simulink model "xpcrs232bindemo"  (Simulink 4.00)
settings: Solver=ode5  StartTime=0.0  StopTime=inf  FixedStep=0.01  RelTol=1e-3
undefined symbols (not defined in the file or in its folder): mrs232
libraries: xpclib x5, simulink3 x1
settings Model: Creator=rroy  LastModifiedBy=rroy  RTWSystemTargetFile=xpctarget.tlc  RTWOptions="-aEnforceIntegerDowncast=0 -aExtMode=1 -aFoldNonRolledExpr=0 -aForceParamTrailComments=0 -aGenerateComments=1 -aIncHierarchyInIds=0 -aInlineInvariantSignals=0 -aInlineParameters=0 -aLocalBlockOutputs=0 -aRL32IRQSourceModifier=\"Timer\" -aRL32LogBufSizeModifier=100000 -aRL32LogTETModifier=1 -aRL32ModeModifier=\"Real-Time\" -aRL32ObjectName=\"tg\" -aRL32ScopeModifier=1 -aRTWVerbose=1 -aRollThreshold=5 -aShowEliminatedStatements=1"  RTWTemplateMakefile=xpc_default_tmf  ExtModeMexFile=ext_xpc  ExtModeArmWhenConnect=off  OptimizeBlockIOStorage=off

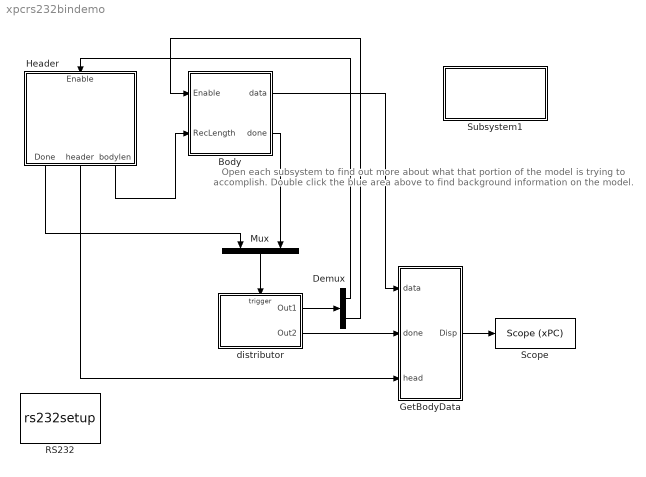
== system xpcrs232bindemo ==
  note: Open each subsystem to find out more
      | about what that portion of the model
      | is trying to accomplish.
      | Double click the blue area above to find
      | background information on the model.
  Body : Subsystem  TreatAsAtomicUnit=on
      settings: RTWFcnNameOpts=Auto  RTWFileNameOpts=Auto
  Demux : Demux  Outputs=2  BusSelectionMode=off
  GetBodyData : Subsystem
      settings: RTWFcnNameOpts=Auto  RTWFileNameOpts=Auto
  Header : Subsystem  Orientation=down  TreatAsAtomicUnit=on
      settings: RTWFcnNameOpts=Auto  RTWFileNameOpts=Auto
  Mux : Mux  Orientation=down  Inputs=2
  "RS232 " : S-Function  AncestorBlock=xpclib/RS232/RS232  InitFcn=mrs232(0);  FunctionName=rs232setup  Parameters=port, baud, dbits, sbits, parity, prot, sbuf, rbuf, 0, istr, iack, iackto, tstr, tack, tackto, initinfo, initackinfo, terminfo, termackinfo  PortCounts=[]  SFunctionModules=''  mask(rs232setup){port=COM1, baud=115200, dbits=8, sbits=1, parity=None, prot=None, sbuf=1024, rbuf=1024, initstruct=[], termstruct=[]}
      mask prompts: baud "Baudrate:"; dbits "Number of Databits:"; sbits "Number of Stopbits:"; prot "Protocol:"; sbuf "Send Buffer Size:"; rbuf "Receive Buffer Size:"; initstruct "Initialization Struct:"; termstruct "Termination Struct:"
      mask help:
      | RS-232
      | Mainboard
      | Setup
      mask init:
      | dmy = '';
      | [istr,iack,dmy,maskdisplay,maskdescription,dmy,dmy,dmy,dmy,initinfo,initackinfo,iackto]=mrs232(2,initstruct,4);
      | [tstr,tack,dmy,maskdisplay,maskdescription,dmy,dmy,dmy,dmy,terminfo,termackinfo,tackto]=mrs232(1,termstruct,4);
      | set_param(gcb,'MaskDisplay',maskdisplay);
      | set_param(gcb,'MaskDescription',maskdescription);
      mask Help: helpview([docroot '/toolbox/xpc/pt_io_block_reference.html#xpcioref'])
      mask StyleString: popup(COM1|COM2|COM3|COM4),popup(115200|57600|38400|19200|9600|4800|2400|1200|600|300|110),popup(8|7),popup(1|2),popup(None|Odd|Even),popup(None|XOn XOff),edit,edit,edit,edit
      mask Display: disp('RS-232\nMainboard\nSetup');
  Scope : xpclib/Misc./Scope (xPC)   scopeno=1  scopetype=Target  viewmode=Numerical  grid=on  ylimits=[0,0]  autostart=on  nosamples=3  noprepostsamples=0  interleave=1  triggermode=FreeRun  triggersignal=1  triggerlevel=0.0  triggerslope=either  triggerscope=1
  Subsystem1 : Subsystem
      settings: OpenFcn=helpview([docroot '\mapfiles\xpc.map'], 'RS232_Binary_Example');  RTWFcnNameOpts=Auto  RTWFileNameOpts=Auto
      mask Display: disp('Double Click\nfor help')
  distributor : Subsystem  TreatAsAtomicUnit=on
      settings: RTWFcnNameOpts=Auto  RTWFileNameOpts=Auto
  wires:
  Body/2(done) -> Mux/2
  Header/3(bodylen) -> Body/2(RecLength)
  distributor/1(Out1) -> Demux/1
  Header/2(header) -> GetBodyData/3(head)
  GetBodyData/1(Disp) -> Scope/1
  Mux/1 -> distributor/Trigger
  Demux/1 -> Header/1(Enable)
  Demux/2 -> Body/1(Enable)
  Body/1(data) -> GetBodyData/1(data)
  distributor/2(Out2) -> GetBodyData/2(done)
  Header/1(Done) -> Mux/1

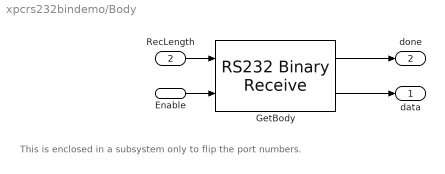
== system xpcrs232bindemo/Body ==
  note: This is enclosed in a subsystem
      | only to flip the port numbers.
  Enable : Inport  Port=1  LatchInput=off
  RecLength : Inport  Port=2  LatchInput=off
  GetBody : xpclib/RS232/Binary Mode/RS232 Binary Receive  port=COM1  width=6  samptime=-1
  data : Outport  Port=1
  done : Outport  Port=2
  wires:
  RecLength/1 -> GetBody/1
  Enable/1 -> GetBody/2
  GetBody/1 -> done/1
  GetBody/2 -> data/1

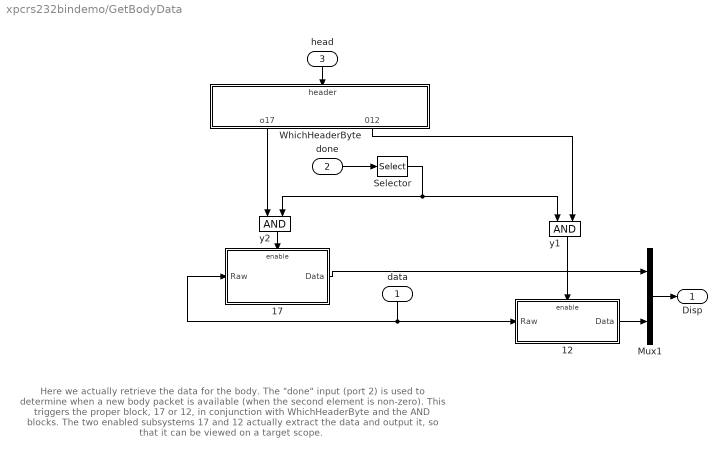
== system xpcrs232bindemo/GetBodyData ==
  note: Here we actually retrieve the data for the body. The "done" input (port 2)
      | is used to determine when a new body packet is available (when the second
      | element is non-zero). This triggers the proper block, 17 or 12, in conjunction
      | with WhichHeaderByte and the AND blocks.
      | The two enabled subsystems 17 and 12 actually extract the data and output
      | it, so that it can be viewed on a target scope.
  data : Inport  Orientation=down  Port=1  LatchInput=off
  done : Inport  Port=2  LatchInput=off
  head : Inport  Orientation=down  Port=3  LatchInput=off
  12 : Subsystem  TreatAsAtomicUnit=on
      settings: RTWFcnNameOpts=Auto  RTWFileNameOpts=Auto
  17 : Subsystem  TreatAsAtomicUnit=on
      settings: RTWFcnNameOpts=Auto  RTWFileNameOpts=Auto
  Mux1 : Mux  Inputs=2
  Selector : Selector  InputType=Vector  ElementSrc=Internal  Elements=2  RowSrc=Internal  Rows=1  ColumnSrc=Internal  Columns=1  InputPortWidth=2
  WhichHeaderByte : Subsystem  Orientation=down
      settings: RTWFcnNameOpts=Auto  RTWFileNameOpts=Auto
  y1 : Logic  Orientation=down  Operator=AND  Inputs=2
  y2 : Logic  Orientation=down  Operator=AND  Inputs=2
  Disp : Outport  Port=1
  wires:
  17/1(Data) -> Mux1/1
  12/1(Data) -> Mux1/2
  head/1 -> WhichHeaderByte/1(header)
  Mux1/1 -> Disp/1
  data/1 -> 17/1(Raw), 12/1(Raw)
  y1/1 -> 12/Enable
  WhichHeaderByte/1(o17) -> y2/1
  y2/1 -> 17/Enable
  WhichHeaderByte/2(012) -> y1/2
  done/1 -> Selector/1
  Selector/1 -> y1/1, y2/2

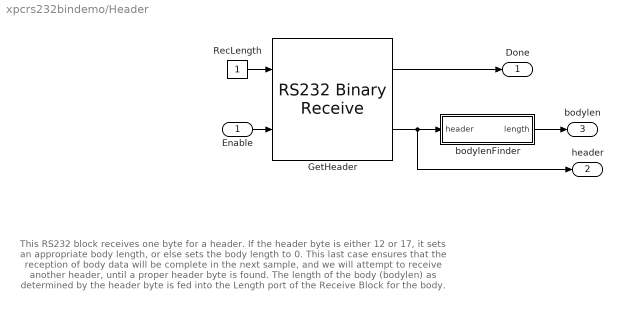
== system xpcrs232bindemo/Header ==
  note: This RS232 block receives one byte for a header.
      | If the header byte is either 12 or 17, it sets an appropriate
      | body length, or else sets the body length to 0. This last case
      | ensures that the reception of body data will be complete in
      | the next sample, and we will attempt to receive another
      | header, until a proper header byte is found.
      | The length of the body (bodylen) as determined by the
      | header byte is fed into the Length port of the Receive
      | Block for the body.
  Enable : Inport  Port=1  LatchInput=off
  GetHeader : xpclib/RS232/Binary Mode/RS232 Binary Receive  port=COM1  width=1  samptime=-1
  RecLength : Constant  Value=1
  bodylenFinder : Subsystem
      settings: RTWFcnNameOpts=Auto  RTWFileNameOpts=Auto
  Done : Outport  Port=1
  header : Outport  Port=2
  bodylen : Outport  Port=3
  wires:
  Enable/1 -> GetHeader/2
  RecLength/1 -> GetHeader/1
  bodylenFinder/1(length) -> bodylen/1
  GetHeader/1 -> Done/1
  GetHeader/2 -> bodylenFinder/1(header), header/1

== system xpcrs232bindemo/Subsystem1 ==

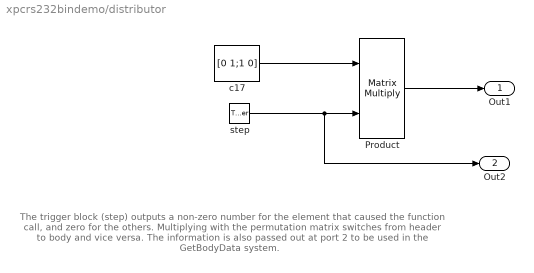
== system xpcrs232bindemo/distributor ==
  note: The trigger block (step) outputs a non-zero number for
      | the element that caused the function call, and zero for
      | the others. Multiplying with the permutation matrix switches
      | from header to body and vice versa. The information is
      | also passed out at port 2 to be used in the GetBodyData
      | system.
  step : TriggerPort  TriggerType=function-call  ShowOutputPort=on  OutputDataType=double
  Product : Product  Inputs=2  Multiplication=Matrix(*)  SaturateOnIntegerOverflow=on
  c17 : Constant  Value=[0 1;1 0]
  Out1 : Outport  Port=1  InitialOutput=[1 0]
  Out2 : Outport  Port=2  InitialOutput=[1 0]
  wires:
  step/1 -> Product/2, Out2/1
  c17/1 -> Product/1
  Product/1 -> Out1/1

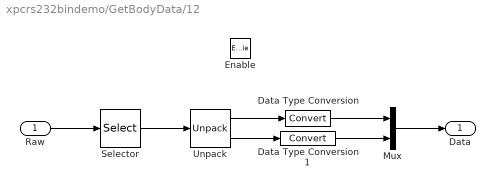
== system xpcrs232bindemo/GetBodyData/12 ==
  Raw : Inport  Port=1  LatchInput=off
  Enable : EnablePort
  Data Type Conversion : DataTypeConversion  DataType=double  SaturateOnIntegerOverflow=on
  Data Type Conversion1 : DataTypeConversion  DataType=double  SaturateOnIntegerOverflow=on
  Mux : Mux  Inputs=2
  Selector : Selector  InputType=Vector  ElementSrc=Internal  Elements=[1:4]  RowSrc=Internal  Rows=1  ColumnSrc=Internal  Columns=1  InputPortWidth=6
  Unpack : xpclib/UDP/Unpack  dimensions={1,1}  datatypes={'uint16', 'int16'}  byteAlign=1
  Data : Outport  Port=1
  wires:
  Raw/1 -> Selector/1
  Unpack/1 -> Data Type Conversion/1
  Unpack/2 -> Data Type Conversion1/1
  Selector/1 -> Unpack/1
  Data Type Conversion/1 -> Mux/1
  Data Type Conversion1/1 -> Mux/2
  Mux/1 -> Data/1

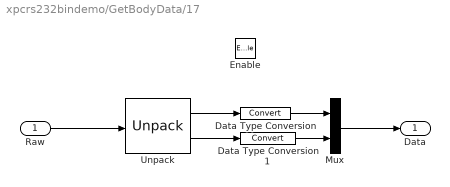
== system xpcrs232bindemo/GetBodyData/17 ==
  Raw : Inport  Port=1  LatchInput=off
  Enable : EnablePort
  Data Type Conversion : DataTypeConversion  DataType=double  SaturateOnIntegerOverflow=on
  Data Type Conversion1 : DataTypeConversion  DataType=double  SaturateOnIntegerOverflow=on
  Mux : Mux  Inputs=2
  Unpack : xpclib/UDP/Unpack  dimensions={1,1}  datatypes={'uint16','int32'}  byteAlign=1
  Data : Outport  Port=1
  wires:
  Unpack/1 -> Data Type Conversion/1
  Unpack/2 -> Data Type Conversion1/1
  Data Type Conversion/1 -> Mux/1
  Data Type Conversion1/1 -> Mux/2
  Mux/1 -> Data/1
  Raw/1 -> Unpack/1

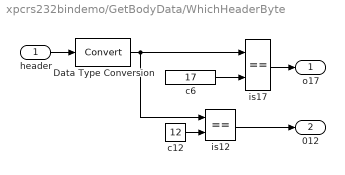
== system xpcrs232bindemo/GetBodyData/WhichHeaderByte ==
  header : Inport  Port=1  LatchInput=off
  Data Type Conversion : DataTypeConversion  DataType=double  SaturateOnIntegerOverflow=on
  c12 : Constant  Value=12
  c6 : Constant  Value=17
  is12 : RelationalOperator  Operator===
  is17 : RelationalOperator  Operator===
  o17 : Outport  Port=1
  012 : Outport  Port=2
  wires:
  is12/1 -> 012/1
  is17/1 -> o17/1
  c12/1 -> is12/2
  c6/1 -> is17/2
  header/1 -> Data Type Conversion/1
  Data Type Conversion/1 -> is12/1, is17/1

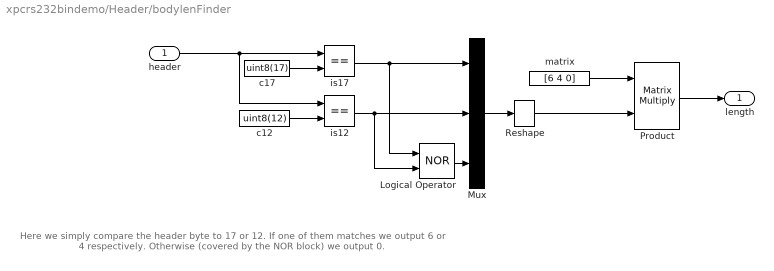
== system xpcrs232bindemo/Header/bodylenFinder ==
  note: Here we simply compare the header byte to 17 or 12.
      | If one of them matches we output 6 or 4 respectively.
      | Otherwise (covered by the NOR block) we output 0.
  header : Inport  Port=1  LatchInput=off
  Logical Operator : Logic  Operator=NOR  Inputs=2
  Mux : Mux  Inputs=3
  Product : Product  Inputs=2  Multiplication=Matrix(*)  SaturateOnIntegerOverflow=on
  Reshape : simulink3/Signals & Systems/Reshape  OutputDimensionality=Column vector  OutputDimensions=[1,1]
  c12 : Constant  Value=uint8(12)
  c17 : Constant  Value=uint8(17)
  is12 : RelationalOperator  Operator===
  is17 : RelationalOperator  Operator===
  matrix : Constant  Value=[6 4 0]  VectorParams1D=off
  length : Outport  Port=1
  wires:
  c17/1 -> is17/2
  c12/1 -> is12/2
  matrix/1 -> Product/1
  is17/1 -> Mux/1, Logical Operator/1
  is12/1 -> Mux/2, Logical Operator/2
  Mux/1 -> Reshape/1
  Product/1 -> length/1
  Reshape/1 -> Product/2
  header/1 -> is17/1, is12/1
  Logical Operator/1 -> Mux/3
